simulink model "siasun_config_casadi_VS_lsj_sim_16a"  (R2019b)
settings: Solver=FixedStepAuto  StartTime=0.0  StopTime=20  FixedStep=0.001  RelTol=1e-3  EnableMultiTasking=on
undefined symbols (not defined in the file): a1, a2, a3, d1, d4, fc1, fc2, fc3, fc4, fc5, fc6, fv1, fv2, fv3, fv4, fv5, fv6, Ia1, Ia2, Ia3, Ia4, Ia5, Ia6, Ic111, Ic112, Ic113, Ic122, Ic123, Ic133, Ic211, Ic212, Ic213, Ic222, Ic223, Ic233, Ic311, Ic312, Ic313, Ic322, Ic323, Ic333, Ic411, Ic412, Ic413, Ic422, Ic423, Ic433, Ic511, Ic512, Ic513, Ic522, Ic523, Ic533, Ic611, Ic612, Ic613, Ic622, Ic623, Ic633, m1 ... (+26)
libraries: sm_lib x224, nesl_utility x124, simulink x8
(part 10 of 10)

== matlab function siasun_config_casadi_VS_lsj_sim_16a/siasun_rel/Robot/Robot/robot/friction ==
  data: u input; y output; fv input; fc input
function y = fcn(u,fv,fc)
%#codegen


% fv1=100; fc1=80; fv2=150; fc2=100; fv3=100; fc3=50; fv4=80; fc4=80; fv5=50; fc5=30; fv6=30; fc6=10;
fv1=fv(1); fc1=fc(1); fv2=fv(2); fc2=fc(2); fv3=fv(3); fc3=fc(3); fv4=fv(4); fc4=fc(4); fv5=fv(5); fc5=fc(5); fv6=fv(6); fc6=fc(6);
y=[0;0;0;0;0;0];
y(1)=(fv1*u(1)+fc1*sign(u(1)));
y(2)=(fv2*u(2)+fc2*sign(u(2)));
y(3)=(fv3*u(3)+fc3*sign(u(3)));
y(4)=(fv4*u(4)+fc4*sign(u(4)));
y(5)=(fv5*u(5)+fc5*sign(u(5)));
y(6)=(fv6*u(6)+fc6*sign(u(6)));

end

== matlab function siasun_config_casadi_VS_lsj_sim_16a/siasun_obs/Robot/Robot/robot/Jm ==
  data: u input; y output; Jm input
function y = fcn(u,Jm)
%#codegen

% Jm=[200; 250; 150; 100; 50; 20];%关节惯性
y = Jm.*u;
end

== matlab function siasun_config_casadi_VS_lsj_sim_16a/siasun_obs/Robot/Robot/robot/friction ==
  data: u input; y output; fv input; fc input
function y = fcn(u,fv,fc)
%#codegen


% fv1=100; fc1=80; fv2=150; fc2=100; fv3=100; fc3=50; fv4=80; fc4=80; fv5=50; fc5=30; fv6=30; fc6=10;
fv1=fv(1); fc1=fc(1); fv2=fv(2); fc2=fc(2); fv3=fv(3); fc3=fc(3); fv4=fv(4); fc4=fc(4); fv5=fv(5); fc5=fc(5); fv6=fv(6); fc6=fc(6);
y=[0;0;0;0;0;0];
y(1)=(fv1*u(1)+fc1*sign(u(1)));
y(2)=(fv2*u(2)+fc2*sign(u(2)));
y(3)=(fv3*u(3)+fc3*sign(u(3)));
y(4)=(fv4*u(4)+fc4*sign(u(4)));
y(5)=(fv5*u(5)+fc5*sign(u(5)));
y(6)=(fv6*u(6)+fc6*sign(u(6)));

end

== matlab function siasun_config_casadi_VS_lsj_sim_16a/DH-CC1 ==
  data: KPS44 input; KPS6 output
function KPS6  = FK(KPS44)
%% parameter
rpy = zeros(1,3);
eps = 0.000001;
%% input 
T=[1 0 0 0;0 1 0 0; 0 0 1 0];
G=KPS44;
H =T * ( G * [0;0;0;1]);
%%
rpy(2) = atan2(-KPS44(3,1),sqrt(KPS44(1,1)*KPS44(1,1)+KPS44(2,1)*KPS44(2,1)));
if (abs(abs(rpy(2)) - pi / 2.0) < eps)
	if (rpy(2) > 0) 
        rpy(2) = pi / 2.0;
        rpy(3) = 0.0;
        rpy(1) = atan2(KPS44(1,2),KPS44(2,2));
    else
    rpy(2) = -pi / 2.0;
	rpy(3) = 0.0;
	rpy(1) = -atan2(KPS44(1,2), KPS44(2,2));
	end
else
	cp = cos(rpy(2));
	rpy(3) = atan2(KPS44(2,1)/cp,KPS44(1,1)/cp);
	rpy(1) = atan2(KPS44(3,2)/cp, KPS44(3,3)/cp);
end
KPS6 = [H' rpy]; 
end

== matlab function siasun_config_casadi_VS_lsj_sim_16a/DH1 ==
  data: Radian input; KPS44 output
function KPS44  = FK(Radian)

%% input 
theta1 = Radian(1);
theta2 = Radian(2);
theta3 = Radian(3);
theta4 = Radian(4);
theta5 = Radian(5);
theta6 = Radian(6);
offset2 = -pi/2; offset3 =0;
Q=[theta1;theta2+offset2;theta3+offset3;theta4;theta5;theta6];
%% D-H parameters 
%XB4
% d1=342;a1=40;a2=275;a3=25;d4=280;dt=73;d3=0;

%siasun
d1=330;a1=40;a2=315;a3=70;d4=324.5;dt=78;d3=0;

%XB7
% d1=380;a1=30;a2=340;a3=35;d4=345;dt=87;d3=0;

Tbase = [1 0 0 0;
        0 1 0 0;
        0 0 1 d1;
        0 0 0 1];
Ttool = [1 0 0 0;
        0 1 0 0;
        0 0 1 dt;
        0 0 0 1];
%% output
II = zeros(4,4);

%% T1~T6
s1=sin(Q(1));s2=sin(Q(2));s3=sin(Q(3));s4=sin(Q(4));s5=sin(Q(5));s6=sin(Q(6));
c1=cos(Q(1));c2=cos(Q(2));c3=cos(Q(3));c4=cos(Q(4));c5=cos(Q(5));c6=cos(Q(6));

t14 = a1*c1 + a3*(c1*c2*c3 - c1*s2*s3) - d3*s1 - d4*(c1*c2*s3 + c1*c3*s2) + a2*c1*c2;
t24 = a1*s1 + c1*d3 + a3*(c2*c3*s1 - s1*s2*s3) - d4*(c2*s1*s3 + c3*s1*s2) + a2*c2*s1;
t34 =-a2*s2 - a3*(c2*s3 + c3*s2) - d4*(c2*c3 - s2*s3);

t11 =s6*(c4*s1 - s4*(c1*c2*c3 - c1*s2*s3)) - c6*(s5*(c1*c2*s3 + c1*c3*s2) - c5*(s1*s4 + c4*(c1*c2*c3 - c1*s2*s3)));
t21 = - c6*(s5*(c2*s1*s3 + c3*s1*s2) + c5*(c1*s4 - c4*(c2*c3*s1 - s1*s2*s3))) - s6*(c1*c4 + s4*(c2*c3*s1 - s1*s2*s3));
t31 = s4*s6*(c2*s3 + c3*s2) - c6*(s5*(c2*c3 - s2*s3) + c4*c5*(c2*s3 + c3*s2));
t12 = s6*(s5*(c1*c2*s3 + c1*c3*s2) - c5*(s1*s4 + c4*(c1*c2*c3 - c1*s2*s3))) + c6*(c4*s1 - s4*(c1*c2*c3 - c1*s2*s3));
t22 =s6*(s5*(c2*s1*s3 + c3*s1*s2) + c5*(c1*s4 - c4*(c2*c3*s1 - s1*s2*s3))) - c6*(c1*c4 + s4*(c2*c3*s1 - s1*s2*s3));
t32 =s6*(s5*(c2*c3 - s2*s3) + c4*c5*(c2*s3 + c3*s2)) + c6*s4*(c2*s3 + c3*s2);
t13= - c5*(c1*c2*s3 + c1*c3*s2) - s5*(s1*s4 + c4*(c1*c2*c3 - c1*s2*s3));
t23 = s5*(c1*s4 - c4*(c2*c3*s1 - s1*s2*s3)) - c5*(c2*s1*s3 + c3*s1*s2);
t33 = c4*s5*(c2*s3 + c3*s2) - c5*(c2*c3 - s2*s3);


II = [t11 t12 t13 t14;
         t21 t22 t23 t24;
         t31 t32 t33 t34;
         0 0 0 1];
     
KPS44 = Tbase*II*Ttool;

end

== matlab function siasun_config_casadi_VS_lsj_sim_16a/xb4_obs/Robot/Robot/robot/Jm ==
  data: u input; y output; Jm input
function y = fcn(u,Jm)
%#codegen

% Jm=[200; 250; 150; 100; 50; 20];%关节惯性
y = Jm.*u;
end

== matlab function siasun_config_casadi_VS_lsj_sim_16a/xb4_obs/Robot/Robot/robot/friction ==
  data: u input; y output; fv input; fc input
function y = fcn(u,fv,fc)
%#codegen


% fv1=100; fc1=80; fv2=150; fc2=100; fv3=100; fc3=50; fv4=80; fc4=80; fv5=50; fc5=30; fv6=30; fc6=10;
fv1=fv(1); fc1=fc(1); fv2=fv(2); fc2=fc(2); fv3=fv(3); fc3=fc(3); fv4=fv(4); fc4=fc(4); fv5=fv(5); fc5=fc(5); fv6=fv(6); fc6=fc(6);
y=[0;0;0;0;0;0];
y(1)=(fv1*u(1)+fc1*sign(u(1)));
y(2)=(fv2*u(2)+fc2*sign(u(2)));
y(3)=(fv3*u(3)+fc3*sign(u(3)));
y(4)=(fv4*u(4)+fc4*sign(u(4)));
y(5)=(fv5*u(5)+fc5*sign(u(5)));
y(6)=(fv6*u(6)+fc6*sign(u(6)));

end

== matlab function siasun_config_casadi_VS_lsj_sim_16a/DH-IK4 ==
  data: angle1 input; t input; Radian output; angle2 input
function Radian  = read(angle1,t,angle2)
if t <= 5
    Radian = angle2;
else
    Radian = angle1;
end
end

== matlab function siasun_config_casadi_VS_lsj_sim_16a/三阶曲线规划1/一关节/3_planning1 ==
  data: state output; plan3_A output; g_vs parameter; g_ve parameter; S input; tf input; tf output
function [state, plan3_A,tf] =planning3( g_vs, g_ve,S,tf)
% 三次多项式算法主程序
% vs初始速度m/min,ve末速度m/min,S总位移m,
% 基础插补规划函数
% 三次多项式速度规划
    a0 = 0 ;
    a1 = g_vs ;
    a2 = 3*S/tf^2 - 2* g_vs/tf - g_ve/tf;
    a3 = -2*S/tf^3 - (g_vs+g_ve)/tf^2;
    state = 1;
    plan3_A = [a0 a1 a2 a3];
    tf =tf ;

end

== matlab function siasun_config_casadi_VS_lsj_sim_16a/三阶曲线规划1/一关节/Interpolation3 ==
  data: state output; Enable input; Y output; plan3_A input; tf input; t input
function [state, Y]  = Interpolate3(Enable,plan3_A,tf,t)
%% input
a0 = plan3_A(1);
a1 = plan3_A(2);
a2 = plan3_A(3);
a3 = plan3_A(4);
Y = 0;
%% output
if Enable == 1
    if t <=tf
    Y = a0 + a1*t + a2*t^2 + a3*t^3; 
    state =1;
    else
    Y = a0 + a1*tf + a2*tf^2 + a3*tf^3;
    state = 1;
    end
else 
    Y = 0;
    state = 0;
end
end

== matlab function siasun_config_casadi_VS_lsj_sim_16a/三阶曲线规划1/三关节/3_planning1 ==
  data: state output; plan3_A output; g_vs parameter; g_ve parameter; S input; tf input; tf output
function [state, plan3_A,tf] =planning3( g_vs, g_ve,S,tf)
% 三次多项式算法主程序
% vs初始速度m/min,ve末速度m/min,S总位移m,
% 基础插补规划函数
% 三次多项式速度规划
    a0 = 0 ;
    a1 = g_vs ;
    a2 = 3*S/tf^2 - 2* g_vs/tf - g_ve/tf;
    a3 = -2*S/tf^3 - (g_vs+g_ve)/tf^2;
    state = 1;
    plan3_A = [a0 a1 a2 a3];
    tf =tf ;

end

== matlab function siasun_config_casadi_VS_lsj_sim_16a/三阶曲线规划1/二关节/3_planning1 ==
  data: state output; plan3_A output; g_vs parameter; g_ve parameter; S input; tf input; tf output
function [state, plan3_A,tf] =planning3( g_vs, g_ve,S,tf)
% 三次多项式算法主程序
% vs初始速度m/min,ve末速度m/min,S总位移m,
% 基础插补规划函数
% 三次多项式速度规划
    a0 = 0 ;
    a1 = g_vs ;
    a2 = 3*S/tf^2 - 2* g_vs/tf - g_ve/tf;
    a3 = -2*S/tf^3 - (g_vs+g_ve)/tf^2;
    state = 1;
    plan3_A = [a0 a1 a2 a3];
    tf =tf ;

end

== matlab function siasun_config_casadi_VS_lsj_sim_16a/三阶曲线规划1/二关节/Interpolation3 ==
  data: state output; Enable input; Y output; plan3_A input; tf input; t input
function [state, Y]  = Interpolate3(Enable,plan3_A,tf,t)
%% input
a0 = plan3_A(1);
a1 = plan3_A(2);
a2 = plan3_A(3);
a3 = plan3_A(4);
Y = 0;
%% output
if Enable == 1
    if t <=tf
    Y = a0 + a1*t + a2*t^2 + a3*t^3; 
    state =1;
    else
    Y = a0 + a1*tf + a2*tf^2 + a3*tf^3;
    state = 1;
    end
else 
    Y = 0;
    state = 0;
end
end

== matlab function siasun_config_casadi_VS_lsj_sim_16a/三阶曲线规划1/五关节/3_planning1 ==
  data: state output; plan3_A output; g_vs parameter; g_ve parameter; S input; tf input; tf output
function [state, plan3_A,tf] =planning3( g_vs, g_ve,S,tf)
% 三次多项式算法主程序
% vs初始速度m/min,ve末速度m/min,S总位移m,
% 基础插补规划函数
% 三次多项式速度规划
    a0 = 0 ;
    a1 = g_vs ;
    a2 = 3*S/tf^2 - 2* g_vs/tf - g_ve/tf;
    a3 = -2*S/tf^3 - (g_vs+g_ve)/tf^2;
    state = 1;
    plan3_A = [a0 a1 a2 a3];
    tf =tf ;

end

== matlab function siasun_config_casadi_VS_lsj_sim_16a/三阶曲线规划1/三关节/Interpolation3 ==
  data: state output; Enable input; Y output; plan3_A input; tf input; t input
function [state, Y]  = Interpolate3(Enable,plan3_A,tf,t)
%% input
a0 = plan3_A(1);
a1 = plan3_A(2);
a2 = plan3_A(3);
a3 = plan3_A(4);
Y = 0;
%% output
if Enable == 1
    if t <=tf
    Y = a0 + a1*t + a2*t^2 + a3*t^3; 
    state =1;
    else
    Y = a0 + a1*tf + a2*tf^2 + a3*tf^3;
    state = 1;
    end
else 
    Y = 0;
    state = 0;
end
end

== matlab function siasun_config_casadi_VS_lsj_sim_16a/三阶曲线规划1/五关节/Interpolation3 ==
  data: state output; Enable input; Y output; plan3_A input; tf input; t input
function [state, Y]  = Interpolate3(Enable,plan3_A,tf,t)
%% input
a0 = plan3_A(1);
a1 = plan3_A(2);
a2 = plan3_A(3);
a3 = plan3_A(4);
Y = 0;
%% output
if Enable == 1
    if t <=tf
    Y = a0 + a1*t + a2*t^2 + a3*t^3; 
    state =1;
    else
    Y = a0 + a1*tf + a2*tf^2 + a3*tf^3;
    state = 1;
    end
else 
    Y = 0;
    state = 0;
end
end

== matlab function siasun_config_casadi_VS_lsj_sim_16a/三阶曲线规划1/六关节/3_planning1 ==
  data: state output; plan3_A output; g_vs parameter; g_ve parameter; S input; tf input; tf output
function [state, plan3_A,tf] =planning3( g_vs, g_ve,S,tf)
% 三次多项式算法主程序
% vs初始速度m/min,ve末速度m/min,S总位移m,
% 基础插补规划函数
% 三次多项式速度规划
    a0 = 0 ;
    a1 = g_vs ;
    a2 = 3*S/tf^2 - 2* g_vs/tf - g_ve/tf;
    a3 = -2*S/tf^3 - (g_vs+g_ve)/tf^2;
    state = 1;
    plan3_A = [a0 a1 a2 a3];
    tf =tf ;

end

== matlab function siasun_config_casadi_VS_lsj_sim_16a/三阶曲线规划1/六关节/Interpolation3 ==
  data: state output; Enable input; Y output; plan3_A input; tf input; t input
function [state, Y]  = Interpolate3(Enable,plan3_A,tf,t)
%% input
a0 = plan3_A(1);
a1 = plan3_A(2);
a2 = plan3_A(3);
a3 = plan3_A(4);
Y = 0;
%% output
if Enable == 1
    if t <=tf
    Y = a0 + a1*t + a2*t^2 + a3*t^3; 
    state =1;
    else
    Y = a0 + a1*tf + a2*tf^2 + a3*tf^3;
    state = 1;
    end
else 
    Y = 0;
    state = 0;
end
end

== matlab function siasun_config_casadi_VS_lsj_sim_16a/三阶曲线规划1/四关节/3_planning1 ==
  data: state output; plan3_A output; g_vs parameter; g_ve parameter; S input; tf input; tf output
function [state, plan3_A,tf] =planning3( g_vs, g_ve,S,tf)
% 三次多项式算法主程序
% vs初始速度m/min,ve末速度m/min,S总位移m,
% 基础插补规划函数
% 三次多项式速度规划
    a0 = 0 ;
    a1 = g_vs ;
    a2 = 3*S/tf^2 - 2* g_vs/tf - g_ve/tf;
    a3 = -2*S/tf^3 - (g_vs+g_ve)/tf^2;
    state = 1;
    plan3_A = [a0 a1 a2 a3];
    tf =tf ;

end

== matlab function siasun_config_casadi_VS_lsj_sim_16a/三阶曲线规划1/四关节/Interpolation3 ==
  data: state output; Enable input; Y output; plan3_A input; tf input; t input
function [state, Y]  = Interpolate3(Enable,plan3_A,tf,t)
%% input
a0 = plan3_A(1);
a1 = plan3_A(2);
a2 = plan3_A(3);
a3 = plan3_A(4);
Y = 0;
%% output
if Enable == 1
    if t <=tf
    Y = a0 + a1*t + a2*t^2 + a3*t^3; 
    state =1;
    else
    Y = a0 + a1*tf + a2*tf^2 + a3*tf^3;
    state = 1;
    end
else 
    Y = 0;
    state = 0;
end
end
